simulink model "svm_sim_singleUAS"  (Simulink 8.6)
settings: Solver=ode1  StartTime=0.0  StopTime=svm.tsim  FixedStep=uavsim.svm.tsample_model  RelTol=1e-6
values from neighbouring files (symbols this model uses):
  My_3D = ([eye(6) -eye(6)])    [svm_buildLinearControllers.m]    (also in svm_setup.m = [-eye(6) eye(6)])
  turbulence2loadfactors = blkdiag(T_w2nx, T_w2nz)    [svm_buildLinearControllers.m]
  uavsim = loaded.uavsim    [svm_sandbox.m]
undefined symbols (not defined in the file or in its folder): F, Light, MIL, postracking, sigbuilder_block, svm, uavsimblockset_cartesianToAngle
libraries: svm_lib x4, aerolibtransform2 x3, uavsimBlockset_UAV3DInterface x2, aerolibwind2 x1, aerolibgravity2 x1, uavsimBlockset_VectorNorm x1, aerolibanimutils x1
settings Model: Creator=j.bolting  LastModifiedBy=j.bolting
settings SolverCC: AutoInsertRateTranBlk=on
settings DataIOCC: SaveFormat=Dataset  SignalLoggingSaveFormat=Dataset
settings OptimizationCC: ExpressionDepthLimit=128
settings DebuggingCC: UnderspecifiedInitializationDetection=Simplified  MergeDetectMultiDrivingBlocksExec=error  SolverPrmCheckMsg=none  FcnCallInpInsideContextMsg=EnableAllAsError  StateNameClashWarn=none
settings HardwareCC: ProdBitPerPointer=64  ProdLargestAtomicFloat=Float  ProdIntDivRoundTo=Zero  ProdEndianess=LittleEndian  ProdWordSize=64  ProdHWDeviceType=Intel->x86-64 (Windows64)
settings GRTTargetCC: GeneratePreprocessorConditionals=Use local settings  CombineOutputUpdateFcns=on  GRTInterface=off
settings ConfigComp: CovModelRefEnable=off

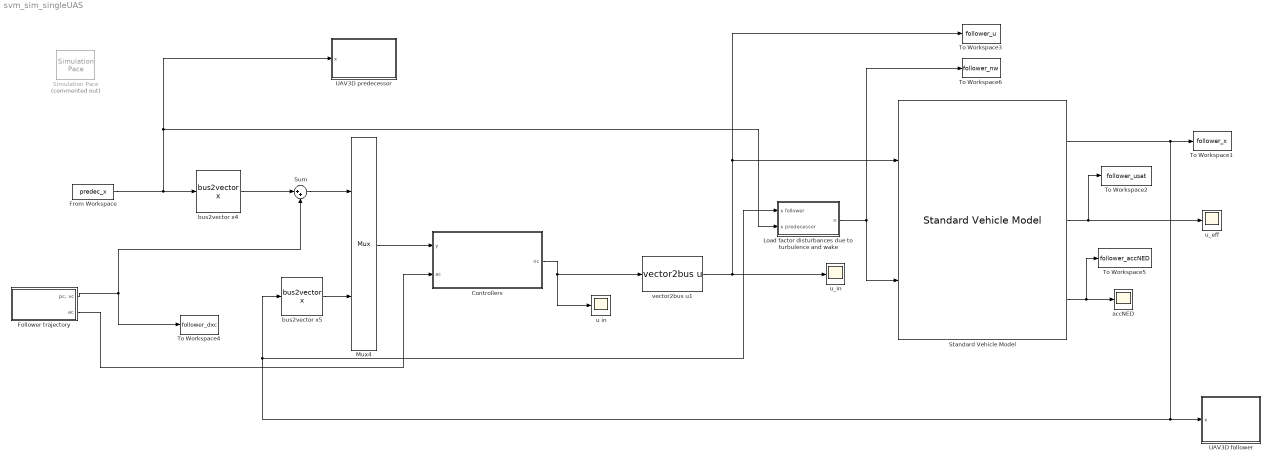
== system svm_sim_singleUAS ==
  Controllers : Subsystem
  Follower trajectory : Subsystem
  From Workspace : FromWorkspace  VariableName=predec_x  OutDataTypeStr=Bus: svm_bus_x
  Load factor disturbances due to turbulence and wake : Subsystem  AncestorBlock=svm_lib/Load factor disturbances due to turbulence
  Mux4 : Mux  Inputs=2
  Simulation Pace : aerolibanimutils/Simulation Pace  Commented=on  SimulationPace=1  SleepMode=MATLAB Thread  OutputPaceError=on  SampleTime=-1
      settings: AttributesFormatString=%<SimulationPace> sec/sec
  Standard Vehicle Model : svm_lib/Standard Vehicle Model  mask_p0_NED=svm.p0  mask_v0_NED=svm.v0
  Sum : Sum  Inputs=|++
  To Workspace1 : ToWorkspace  VariableName=follower_x  SaveFormat=Timeseries  SampleTime=-1
  To Workspace2 : ToWorkspace  VariableName=follower_usat  SaveFormat=Timeseries  SampleTime=-1
  To Workspace3 : ToWorkspace  VariableName=follower_u  SaveFormat=Timeseries  SampleTime=-1
  To Workspace4 : ToWorkspace  VariableName=follower_dxc  SaveFormat=Timeseries  SampleTime=-1
  To Workspace5 : ToWorkspace  VariableName=follower_accNED  SaveFormat=Timeseries  SampleTime=-1
  To Workspace6 : ToWorkspace  VariableName=follower_nw  SaveFormat=Timeseries  SampleTime=-1
  UAV3D follower : Subsystem
  UAV3D predecessor : Subsystem
  accNED : Scope
  bus2vector x4 : svm_lib/bus2vector x
  bus2vector x5 : svm_lib/bus2vector x
  u in : Scope
  u_eff : Scope
  u_in : Scope
  vector2bus u1 : svm_lib/vector2bus u
  wires:
  Standard Vehicle Model/1 -> UAV3D follower/1(x), bus2vector x5/1, Load factor disturbances due to turbulence and wake/1(x follower), To Workspace1/1
  bus2vector x4/1 -> Sum/1
  bus2vector x5/1 -> Mux4/2
  vector2bus u1/1 -> To Workspace3/1, Standard Vehicle Model/1, u_in/1
  From Workspace/1 -> bus2vector x4/1, Load factor disturbances due to turbulence and wake/2(x predecessor), UAV3D predecessor/1(x)
  Controllers/1(nc) -> vector2bus u1/1, u in/1
  Mux4/1 -> Controllers/1(y)
  Load factor disturbances due to turbulence and wake/1(n) -> Standard Vehicle Model/2, To Workspace6/1
  Standard Vehicle Model/2 -> u_eff/1, To Workspace2/1
  Standard Vehicle Model/3 -> accNED/1, To Workspace5/1
  Sum/1 -> Mux4/1
  Follower trajectory/1("pc, vc") -> To Workspace4/1, Sum/2
  Follower trajectory/2(ac) -> Controllers/2(ac)

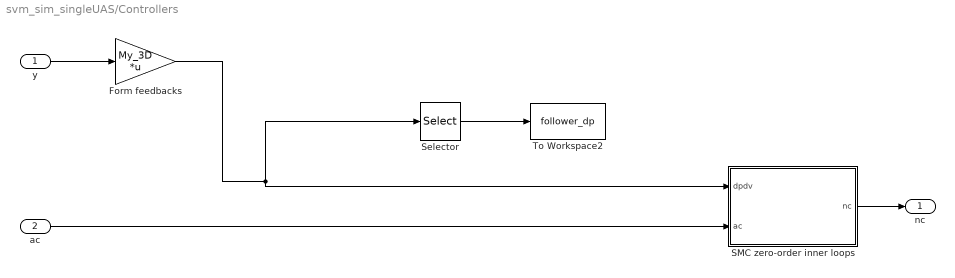
== system svm_sim_singleUAS/Controllers ==
  y : Inport
  ac : Inport  Port=2
  Form feedbacks : Gain  Gain=My_3D  Multiplication=Matrix(K*u)
  SMC zero-order inner loops : Subsystem
  Selector : Selector  InputPortWidth=6  IndexOptions=Index vector (dialog)  Indices=1:3  OutputSizes=1
  To Workspace2 : ToWorkspace  VariableName=follower_dp  SaveFormat=Timeseries  SampleTime=-1
  nc : Outport
  wires:
  SMC zero-order inner loops/1(nc) -> nc/1
  y/1 -> Form feedbacks/1
  Form feedbacks/1 -> Selector/1, SMC zero-order inner loops/1(dpdv)
  ac/1 -> SMC zero-order inner loops/2(ac)
  Selector/1 -> To Workspace2/1

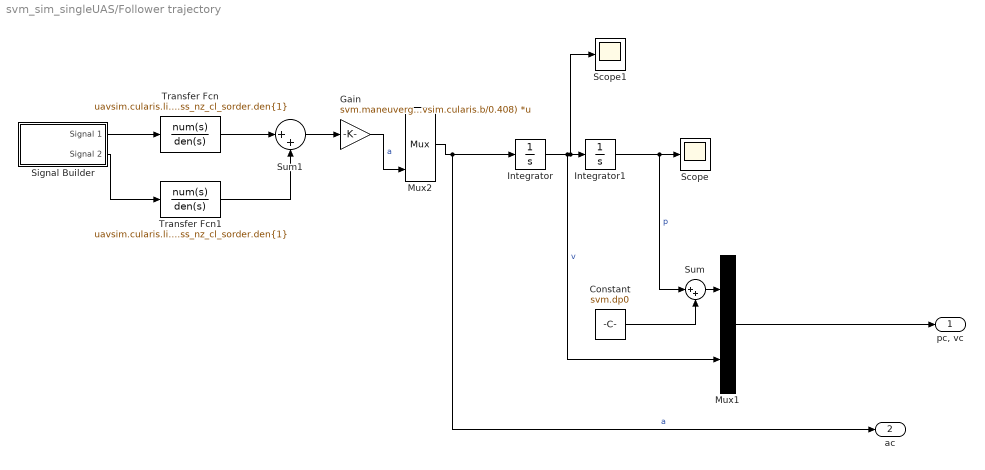
== system svm_sim_singleUAS/Follower trajectory ==
  Constant : Constant  Value=svm.dp0
  Gain : Gain  Gain=svm.maneuvergain*4*(1*uavsim.cularis.b/0.408)  Multiplication=Matrix(K*u)
  Integrator : Integrator
  Integrator1 : Integrator
  Mux1 : Mux  Inputs=2
  Mux2 : Mux  Inputs=3
  Scope : Scope
  Scope1 : Scope
  Signal Builder : Subsystem  Tag=STV Subsys  LoadFcn=sigbuilder_block('load');  StartFcn=sigbuilder_block('start');  StopFcn=sigbuilder_block('stop');  ClipboardFcn=sigbuilder_block('clipboard');  mask(Sigbuilder block){}
      mask help: Simulink:masks:SigbuilderBlock_MD
      mask init:
      | if ~strcmp(get_param(bdroot(gcbh),'SimulationStatus'),'stopped') tuvar = sigbuilder_block('maskInit'); end
      settings: CopyFcn=sigbuilder_block('copy');  DeleteFcn=sigbuilder_block('delete');  ModelCloseFcn=sigbuilder_block('modelClose');  PreSaveFcn=sigbuilder_block('preSave');  PauseFcn=sigbuilder_block('pause');  ContinueFcn=sigbuilder_block('continue');  NameChangeFcn=sigbuilder_block('namechange');  OpenFcn=sigbuilder_block('open',[219.6 199.2 768.6 400.2 ]);  CloseFcn=sigbuilder_block('close');
      mask Display: plot(0, 0, 100, 100,[2, 2, 32, 32, 2], [68, 8, 8, 68, 68],[32, 2], [38, 38], [32, 19, 2],[53, 60, 44], [32, 17, 17, 2],[16, 16, 31, 31]);txt = getActiveGroup(gcbh);text(2, 100, txt,'verticalAlignment', 'top');
  Sum : Sum  Inputs=|++
  Sum1 : Sum  Inputs=|++
  Transfer Fcn : TransferFcn  Numerator=uavsim.cularis.linearModels.eulers.ss_nz_cl_sorder.num{1}  Denominator=uavsim.cularis.linearModels.eulers.ss_nz_cl_sorder.den{1}
  Transfer Fcn1 : TransferFcn  Numerator=uavsim.cularis.linearModels.eulers.ss_nz_cl_sorder.num{1}  Denominator=uavsim.cularis.linearModels.eulers.ss_nz_cl_sorder.den{1}
  "pc, vc" : Outport
  ac : Outport  Port=2
  wires:
  Mux1/1 -> "pc, vc"/1
  Signal Builder/1(Signal 1) -> Transfer Fcn/1
  Signal Builder/2(Signal 2) -> Transfer Fcn1/1
  Sum1/1 -> Gain/1
  Transfer Fcn/1 -> Sum1/1
  Transfer Fcn1/1 -> Sum1/2
  Mux2/1 -> ac/1, Integrator/1  "a"
  Integrator/1 -> Mux1/2, Scope1/1, Integrator1/1  "v"
  Integrator1/1 -> Sum/1, Scope/1  "p"
  Sum/1 -> Mux1/1
  Constant/1 -> Sum/2
  Gain/1 -> Mux2/3  "a"

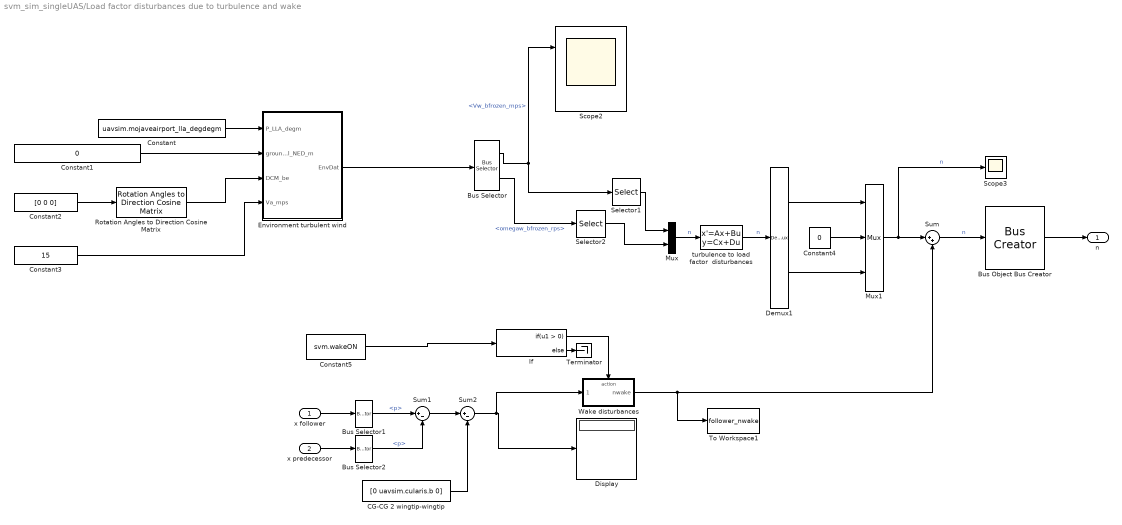
== system svm_sim_singleUAS/Load factor disturbances due to turbulence and wake ==
  x follower : Inport  OutDataTypeStr=Bus: svm_bus_x
  x predecessor : Inport  Port=2  OutDataTypeStr=Bus: svm_bus_x
  Bus Selector : BusSelector  OutputSignals=Vw_bfrozen_mps,omegaw_bfrozen_rps
  Bus Selector1 : BusSelector  OutputSignals=p
  Bus Selector2 : BusSelector  OutputSignals=p
  Bus Object Bus Creator : BusCreator  Inputs=1  OutDataTypeStr=Bus: svm_bus_u  mask(BUS OBJECT Bus Creator){busType=Bus: svm_bus_u}
      mask prompts: busType "Bus Type"
      mask help:
      | Provides users the cabability to painlessly, instantly customize bus creators of output data type 'Bus:' by selecting the bus object type from a drop down menu dynamically populated by bus objects in the workspace.
      |
      | After pressing the "Apply Selection" button signal lines into the creator are populated and named with the elements in the chosen bus saving the user from having to recall and fill out signal line names.
      |
      | NOTE that when copying a Bus Object Bus Creator from your locked Library the link to the Library is automatically broken. This saves the user from having to Unlock Links To Library (From the Library menu.), Disable Link and finally Break Link (Both from the Model menu.) for every placed instance of the block.
      settings: AttributesFormatString=%<OutDataTypeStr>  CopyFcn=set_param(gcb, 'LinkStatus', 'none')
      mask TypeOptions busType: Bus: Acceleration | Bus: Aero | Bus: Airframe | Bus: Attitude | Bus: CMD | Bus: Environment | Bus: FlightGearData | Bus: Kinematics | Bus: Position | Bus: RotationalAcceleration | Bus: RotationalVelocity | Bus: Velocity | Bus: svm_bus_d_exo | Bus: svm_bus_u | Bus: svm_bus_x | Bus: svm_bus_xi
      mask Callback busType:
      | % Using variable names terminated with "_BOBC" to lessen the chances of
      | % collisions with existing workspace variables.
      | 
      | % Get the current block handle and mask handle.
      | handleCreator_BOBC = gcbh;
      | maskObj_BOBC       = Simulink.Mask.get(gcb);
      | 
      | % Get a list of variables in the workspace in order to search for the '1x1
      | % Bus' types.
      | wsVars_BOBC = whos;
      | 
      | % Reset the 'TypeOptions' bus list in case some '1x1 Bus' types have been
      | % deleted from or added to the workspace.
      | maskObj_BOBC.Parameters.TypeOptions = {'<empty>'};
      | 
      | % Reset the bus count.
      | busCount_BOBC = 0;
      | 
      | for index_BOBC = 1:length(wsVars_BOBC)
      | 
      |    % If the variable is a bus object...
      |    if strcmp(wsVars_BOBC(index_BOBC).class, 'Simulink.Bus')
      | 
      |       busCount_BOBC = busCount_BOBC + 1;
      | 
      |       % ... add it to the TypeOptions of the mask.
      |       maskObj_BOBC.Parameters.TypeOptions(busCount_BOBC) = ...
      |                                                            ...
      |                                  {['Bus: ', wsVars_BOBC(index_BOBC).name]};
      |    end
      | end
      | 
      | if busCount_BOBC == 0
      | 
      |    % If there are NO bus objects in the workspace then provide a warning
      |    % popup...
      |    warndlg('There are currently no bus objects in the workspace - you have no use for this block. Use a normal Bus Creator instead.')
      | 
      |    % ... and do nothing.
      | elseif ~strcmp(get_param(handleCreator_BOBC, 'OutDataTypeStr'), 'Inherit: auto')
      | 
      |    % If the currently selected bus data type ('OutDataTypeStr') is not
      |    % 'Inherit: auto' (i.e., if we are reopening the mask.) then get the
      |    % current 'OutDataTypeStr' and 'maskVal.' ('maskVal' is the selected
      |    % 'TypeOptions' list member.)
      |    outDatStr_BOBC = get_param(handleCreator_BOBC, 'OutDataTypeStr');
      |    maskVal_BOBC   = get_param(handleCreator_BOBC, 'MaskValues');
      | 
      |    if ~strcmp(outDatStr_BOBC, maskVal_BOBC{1})
      | 
      |       % Upon re-opening the mask if the default 'TypeOptions' list member
      |       % (The first one.) contained in 'maskVal' does not match the
      |       % currently selected bus data type ('OutDataTypeStr') then set the
      |       % 'TypeOptions' list member to the selected bus data type. (Cuts down
      |       % on confusion to have the displayed list member match the selected
      |       % bus data type rather than the first entry.)
      |       set_param(handleCreator_BOBC, 'MaskValues', {outDatStr_BOBC});
      |    end
      | end
      | 
      | % Clean up the workspace.
      | clear  handleCreator_BOBC  maskObj_BOBC     wsVars_BOBC ...
      |             busCount_BOBC    index_BOBC  outDatStr_BOBC ...
      |              maskVal_BOBC
      mask DialogControl applyMOCBSelection Prompt: Apply Selection
      mask DialogControl applyMOCBSelection Callback:
      | % Using variable names terminated with "_BOBC" to lessen the chances of
      | % collisions with existing workspace variables.
      | 
      | % Get the current block, current block handle and mask handle.
      | currentBlock_BOBC  = gcb;
      | handleCreator_BOBC = gcbh;
      | 
      | % Get the desired bus type...
      | desiredBusType_BOBC = get_param(handleCreator_BOBC, 'busType');
      | 
      | % ... and set the 'OutDataTypeStr' to it.
      | set_param(handleCreator_BOBC, 'OutDataTypeStr', desiredBusType_BOBC);
      | 
      | %% First delete any existing lines on the port.
      | % Get the line handles.
      | lh_BOBC = get_param(handleCreator_BOBC, 'LineHandles');
      | 
      | % If any lines exist (Non- -1 line handles.), delete them and start over.
      | if max(lh_BOBC.Inport > 0)
      | 
      |    for index_BOBC = 1:length(lh_BOBC.Inport)
      | 
      |       if lh_BOBC.Inport(index_BOBC) > 0
      | 
      |          delete_line(lh_BOBC.Inport(index_BOBC))
      |       end
      |    end
      | end
      | 
      | %% Then work on adding new lines.
      | 
      | % Get the block path for 'add_line' function.
      | blockPath_BOBC = get_param(handleCreator_BOBC, 'Parent');
      | 
      | % Get the newly selected bus type ('OutDataTypeStr')...
      | mocbBusType_BOBC = get_param(currentBlock_BOBC, 'OutDataTypeStr');
      | 
      | % ... and parse off "Bus: " so the string of the desired bus contained in
      | % 'OutDataTypeStr' matches the raw workspace bus names.
      | mocbBusType_BOBC = mocbBusType_BOBC(6:end);
      | 
      | % Then evaluate the string containing the workspace bus name which will
      | % load the desired bus parameters.
      | busParams_BOBC = eval(mocbBusType_BOBC);
      | 
      | % From the parameters grab the number of lines to add.
      | numLines_BOBC = length(busParams_BOBC.Elements);
      | 
      | % Set the number of inputs of the masked bus creator to the number of lines
      | % to add.
      | set_param(handleCreator_BOBC, 'Inputs', num2str(numLines_BOBC));
      | 
      | % Get (Inputs.) port handles so we can grab the positions of them.
      | ph_BOBC = get_param(handleCreator_BOBC, 'PortHandles');
      | 
      | for index_BOBC = 1:numLines_BOBC
      | 
      |    % Get the position of input port number 'index_BOBC'.
      |    portPos_BOBC = get_param(ph_BOBC.Inport(index_BOBC), 'Position');
      | 
      |    % Add a line from 50 pixels left of the port position to the port
      |    % position. (This must be done because it's the lines that get named,
      |    % not the port positions.)
      |    portLine_BOBC = add_line(blockPath_BOBC, [portPos_BOBC - [50 0]; portPos_BOBC]);
      | 
      |    % Rename the new line to the bus 'index_BOBC-st/nd/rd/th' element name.
      |    set_param(portLine_BOBC, 'Name', busParams_BOBC.Elements(index_BOBC).Name)
      | end
      | 
      | %% Cleanup the workspace.
      | clear    currentBlock_BOBC  handleCreator_BOBC      index_BOBC ...
      |        desiredBusType_BOBC             lh_BOBC  blockPath_BOBC ...
      |           mocbBusType_BOBC      busParams_BOBC   numLines_BOBC ...
      |                    ph_BOBC        portPos_BOBC   portLine_BOBC
  CG-CG 2 wingtip-wingtip : Constant  Value=[0 uavsim.cularis.b 0]
  Constant : Constant  Value=uavsim.mojaveairport_lla_degdegm
  Constant1 : Constant  Value=0
  Constant2 : Constant  Value=[0 0 0]
  Constant3 : Constant  Value=15
  Constant4 : Constant  Value=0
  Constant5 : Constant  Value=svm.wakeON
  Demux1 : Demux  Outputs=2
  Display : Display
  Environment turbulent wind : Subsystem  AncestorBlock=uavsimBlockset_Environment_turbulentWind/Environment turbulent wind  mask{mask_constantwind_NED_mps=svm.ambientWind, mask_wingspan=uavsim.cularis.b, mask_windON=svm.ambientWindOn, mask_turbulenceON=svm.turbulenceOn}
      mask prompts: mask_constantwind_NED_mps "Ambient, i.e. constant wind vector [m/s], NED frame"; mask_wingspan "Aircraft wingspan"; mask_windON "Ambient wind ON?"; mask_turbulenceON "Turbulence ON?"
  If : If
  Mux : Mux  Inputs=2
  Mux1 : Mux  Inputs=3
  Rotation Angles to Direction Cosine Matrix : aerolibtransform2/Rotation Angles to Direction Cosine Matrix  rotationOrder=ZYX
  Scope2 : Scope  NumInputPorts=2
  Scope3 : Scope
  Selector1 : Selector  InputPortWidth=3  IndexOptions=Index vector (dialog)  Indices=[1 3]  OutputSizes=1
  Selector2 : Selector  InputPortWidth=3  IndexOptions=Index vector (dialog)  Indices=2  OutputSizes=1
  Sum : Sum  Inputs=|++
  Sum1 : Sum  Inputs=|+-
  Sum2 : Sum  Inputs=|+-
  Terminator : Terminator
  To Workspace1 : ToWorkspace  VariableName=follower_nwake  SaveFormat=Timeseries  SampleTime=-1
  Wake disturbances : Subsystem  TreatAsAtomicUnit=on
  turbulence to load factor  disturbances : StateSpace  A=turbulence2loadfactors.a  B=turbulence2loadfactors.b  C=turbulence2loadfactors.c  D=turbulence2loadfactors.d  X0=0
  n : Outport
  wires:
  Constant4/1 -> Mux1/2
  Demux1/2 -> Mux1/3
  Mux1/1 -> Sum/1, Scope3/1  "n"
  Selector2/1 -> Mux/2
  Constant2/1 -> Rotation Angles to Direction Cosine Matrix/1
  turbulence to load factor  disturbances/1 -> Demux1/1  "n"
  Constant1/1 -> Environment turbulent wind/2(groundlevel_NED_m)
  Demux1/1 -> Mux1/1
  Constant/1 -> Environment turbulent wind/1(P_LLA_degm)
  Bus Selector/1 -> Scope2/1, Selector1/1  "<Vw_bfrozen_mps>"
  Rotation Angles to Direction Cosine Matrix/1 -> Environment turbulent wind/3(DCM_be)
  Bus Selector/2 -> Selector2/1  "<omegaw_bfrozen_rps>"
  Environment turbulent wind/1(EnvDat) -> Bus Selector/1
  Constant3/1 -> Environment turbulent wind/4(Va_mps)
  Bus Object Bus Creator/1 -> n/1
  Mux/1 -> turbulence to load factor  disturbances/1  "n"
  Selector1/1 -> Mux/1
  If/1 -> Wake disturbances/Action
  Constant5/1 -> If/1
  If/2 -> Terminator/1
  Wake disturbances/1(nwake) -> Sum/2, To Workspace1/1
  x follower/1 -> Bus Selector1/1
  x predecessor/1 -> Bus Selector2/1
  Bus Selector1/1 -> Sum1/1  "<p>"
  Bus Selector2/1 -> Sum1/2  "<p>"
  Sum2/1 -> Wake disturbances/1(dp_wingtips), Display/1
  CG-CG 2 wingtip-wingtip/1 -> Sum2/2
  Sum1/1 -> Sum2/1
  Sum/1 -> Bus Object Bus Creator/1  "n"

== system svm_sim_singleUAS/UAV3D follower ==
  x : Inport
  Bus Selector5 : BusSelector  OutputSignals=p,v
  Rate Transition10 : RateTransition  OutPortSampleTime=uavsim.svm.tsample_uav3d
  Rate Transition9 : RateTransition  OutPortSampleTime=uavsim.svm.tsample_uav3d
  Vehicle ID2 : Constant  Value=2
  Visualize NED position2 : Subsystem  AncestorBlock=formationFlyingBlockset/Visualize leader  TreatAsAtomicUnit=on  SystemSampleTime=uavsim.svm.tsample_uav3d  mask{mask_3dmodel=1}
      mask prompts: mask_3dmodel "3D model"
      mask TypeOptions mask_3dmodel: 0 | 1 | 2 | 3
  wires:
  x/1 -> Bus Selector5/1
  Bus Selector5/2 -> Rate Transition10/1  "<v>"
  Vehicle ID2/1 -> Visualize NED position2/3(ID)
  Bus Selector5/1 -> Rate Transition9/1  "<p>"
  Rate Transition10/1 -> Visualize NED position2/2(v_NED_mps)
  Rate Transition9/1 -> Visualize NED position2/1(p_NED_m)

== system svm_sim_singleUAS/UAV3D predecessor ==
  x : Inport
  Bus Selector1 : BusSelector  OutputSignals=p,v
  Constant5 : Constant
  Rate Transition5 : RateTransition  OutPortSampleTime=uavsim.svm.tsample_uav3d
  Rate Transition6 : RateTransition  OutPortSampleTime=uavsim.svm.tsample_uav3d
  Visualize NED position1 : Subsystem  AncestorBlock=formationFlyingBlockset/Visualize leader  TreatAsAtomicUnit=on  SystemSampleTime=uavsim.svm.tsample_uav3d  mask{mask_3dmodel=1}
      mask prompts: mask_3dmodel "3D model"
      mask TypeOptions mask_3dmodel: 0 | 1 | 2 | 3
  wires:
  x/1 -> Bus Selector1/1
  Rate Transition5/1 -> Visualize NED position1/1(p_NED_m)
  Constant5/1 -> Visualize NED position1/3(ID)
  Rate Transition6/1 -> Visualize NED position1/2(v_NED_mps)
  Bus Selector1/1 -> Rate Transition5/1  "<p>"
  Bus Selector1/2 -> Rate Transition6/1  "<v>"

== system svm_sim_singleUAS/Controllers/SMC zero-order inner loops ==
  dpdv : Inport
  ac : Inport  Port=2
  CSMC : Subsystem  Commented=on  AncestorBlock=svm_lib/SMC-directforce
  DSMC : Subsystem  AncestorBlock=svm_lib/SMC-directforce
  nc : Outport
  wires:
  DSMC/1(nc) -> nc/1
  dpdv/1 -> CSMC/1(dpdv), DSMC/1(dpdv)
  ac/1 -> DSMC/2(ac)

== system svm_sim_singleUAS/Follower trajectory/Signal Builder ==
  Demux : Demux  Tag=STV Demux  Outputs=2
  FromWs : FromWorkspace  Tag=STV FromWs  VariableName=tuvar  SampleTime=0  SigBuilderData=DataTag0  VnvData=DataTag1
      SigBuilderData=|
      | common.afterFinalStr = 'Extrapolate'
      | common.sampleTime = 0
      | dataSet.timeRange = [0 10]
      | dataSet.name = 'Group 1'
      | sbobj.Groups.Name = 'Group 1'
      | sbobj.Groups.Signals(1).Name = 'Signal 1'
      | sbobj.Groups.Signals(1).XData = [0 5 5 6.02 6.02 10]
      | sbobj.Groups.Signals(1).YData = [0 0 -0.1 -0.1 0 0]
      | sbobj.Groups.Signals(2).Name = 'Signal 2'
      | sbobj.Groups.Signals(2).XData = [0 6 6 7.02 7.02 10]
      | sbobj.Groups.Signals(2).YData = [0 0 0.1 0.1 0 0]
  Signal 1 : Outport  Tag=STV Outport
  Signal 2 : Outport  Tag=STV Outport  Port=2
  wires:
  Demux/1 -> Signal 1/1
  FromWs/1 -> Demux/1
  Demux/2 -> Signal 2/1

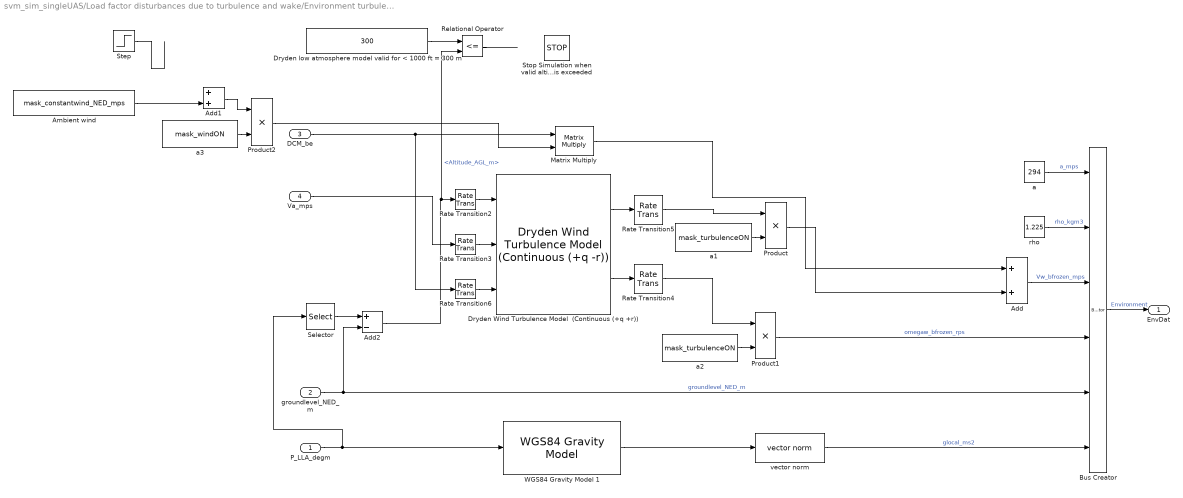
== system svm_sim_singleUAS/Load factor disturbances due to turbulence and wake/Environment turbulent wind ==
  P_LLA_degm : Inport
  groundlevel_NED_m : Inport  Port=2
  DCM_be : Inport  Port=3
  Va_mps : Inport  Port=4
  Add : Sum
  Add1 : Sum
  Add2 : Sum  Inputs=+-
  Ambient wind : Constant  Value=mask_constantwind_NED_mps
  Bus Creator : BusCreator  Inputs=6  OutDataTypeStr=Bus: Environment  NonVirtualBus=on
  Dryden Wind Turbulence Model  (Continuous (+q +r)) : aerolibwind2/Dryden Wind Turbulence Model  (Continuous (+q -r))  units=Metric (MKS)  spec=MIL-F-8785C  model=Discrete Dryden (+q -r)  W20=norm(mask_constantwind_NED_mps)  Wdeg=rad2deg(uavsimblockset_cartesianToAngle(mask_constantwind_NED_mps(1), mask_constantwind_NED_mps(2)))  TurbProb=10^-2 - Light  L_high=533.4  Wingspan=mask_wingspan  ts=uavsim.svm.tsample_dryden  Seed=eval(svm.turbulenceseed)  T_on=on
  Dryden low atmosphere model valid for < 1000 ft = 300 m : Constant  Value=300
  Matrix Multiply : Product  Multiplication=Matrix(*)
  Product : Product  RndMeth=Zero
  Product1 : Product  RndMeth=Zero
  Product2 : Product  RndMeth=Zero
  Rate Transition2 : RateTransition  OutPortSampleTime=uavsim.svm.tsample_dryden
  Rate Transition3 : RateTransition  OutPortSampleTime=uavsim.svm.tsample_dryden
  Rate Transition4 : RateTransition  OutPortSampleTime=0
  Rate Transition5 : RateTransition  OutPortSampleTime=0
  Rate Transition6 : RateTransition  OutPortSampleTime=uavsim.svm.tsample_dryden
  Relational Operator : RelationalOperator  Operator=<=  OutDataTypeStr=boolean
  Selector : Selector  InputPortWidth=3  IndexOptions=Index vector (dialog)  Indices=3  OutputSizes=1
  Step : Step  Time=10  After=[0 0 1]  SampleTime=0
  Stop Simulation when valid altitude is exceeded : Stop
  WGS84 Gravity Model 1 : aerolibgravity2/WGS84 Gravity Model   model=WGS84 Taylor Series  units=Metric (MKS)  no_atmos=on  precessing=on  jd_loc=off  month=October  day=10  year=2004  no_centrifugal=on  action=Warning
  a : Constant  Value=294
  a1 : Constant  Value=mask_turbulenceON
  a2 : Constant  Value=mask_turbulenceON
  a3 : Constant  Value=mask_windON
  "rho " : Constant  Value=1.225
  vector norm : uavsimBlockset_VectorNorm/vector norm
  EnvDat : Outport  OutDataTypeStr=Bus: Environment
  wires:
  Rate Transition6/1 -> Dryden Wind Turbulence Model  (Continuous (+q +r))/3
  Rate Transition3/1 -> Dryden Wind Turbulence Model  (Continuous (+q +r))/2
  Rate Transition2/1 -> Dryden Wind Turbulence Model  (Continuous (+q +r))/1
  Selector/1 -> Add2/1
  Rate Transition5/1 -> Product/1
  Rate Transition4/1 -> Product1/1
  Matrix Multiply/1 -> Add/1
  Dryden Wind Turbulence Model  (Continuous (+q +r))/1 -> Rate Transition5/1
  Ambient wind/1 -> Add1/2
  DCM_be/1 -> Rate Transition6/1, Matrix Multiply/1
  Va_mps/1 -> Rate Transition3/1
  Add2/1 -> Relational Operator/2, Rate Transition2/1  "<Altitude_AGL_m>"
  vector norm/1 -> Bus Creator/6  "glocal_ms2"
  Add/1 -> Bus Creator/3  "Vw_bfrozen_mps"
  a/1 -> Bus Creator/1  "a_mps"
  "rho "/1 -> Bus Creator/2  "rho_kgm3"
  Bus Creator/1 -> EnvDat/1  "Environment"
  WGS84 Gravity Model 1/1 -> vector norm/1
  groundlevel_NED_m/1 -> Bus Creator/5, Add2/2  "groundlevel_NED_m"
  P_LLA_degm/1 -> Selector/1, WGS84 Gravity Model 1/1
  Dryden Wind Turbulence Model  (Continuous (+q +r))/2 -> Rate Transition4/1
  Product/1 -> Add/2
  a1/1 -> Product/2
  a2/1 -> Product1/2
  Product1/1 -> Bus Creator/4  "omegaw_bfrozen_rps"
  Dryden low atmosphere model valid for < 1000 ft = 300 m/1 -> Relational Operator/1
  Relational Operator/1 -> ?
  a3/1 -> Product2/2
  Product2/1 -> Matrix Multiply/2
  Add1/1 -> Product2/1
  Step/1 -> ?

== system svm_sim_singleUAS/Load factor disturbances due to turbulence and wake/Wake disturbances ==
  dp_wingtips : Inport
  Action Port : ActionPort  ActionType=then
  MATLAB Function : MATLAB Function  TreatAsAtomicUnit=on
  nwake : Outport
  wires:
  dp_wingtips/1 -> MATLAB Function/1(dp)
  MATLAB Function/1(nwake) -> nwake/1

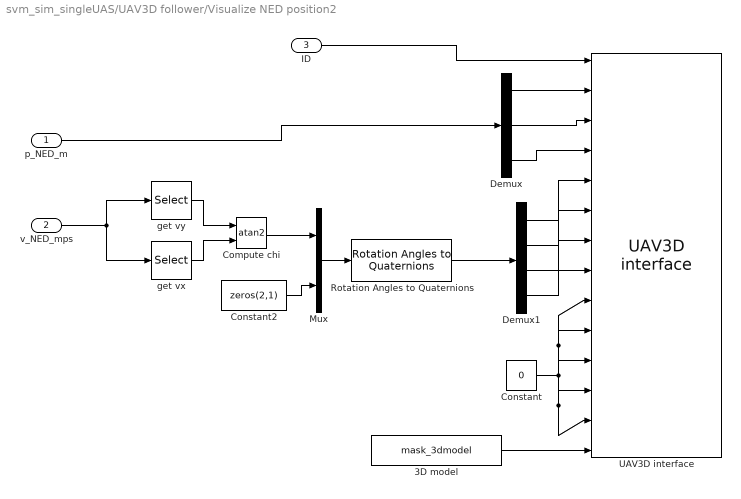
== system svm_sim_singleUAS/UAV3D follower/Visualize NED position2 ==
  p_NED_m : Inport
  v_NED_mps : Inport  Port=2
  ID : Inport  Port=3
  3D model : Constant  Value=mask_3dmodel
  Compute chi : Trigonometry  Operator=atan2
  Constant : Constant  Value=0
  Constant2 : Constant  Value=zeros(2,1)
  Demux : Demux  Outputs=3
  Demux1 : Demux
  Mux : Mux  Inputs=2
  Rotation Angles to Quaternions : aerolibtransform2/Rotation Angles to Quaternions  rotationOrder=ZYX
  UAV3D interface : uavsimBlockset_UAV3DInterface/UAV3D interface  ip='localhost'  udpport=4445
  get vx : Selector  InputPortWidth=3  IndexOptions=Index vector (dialog)  Indices=1  OutputSizes=1
  get vy : Selector  InputPortWidth=3  IndexOptions=Index vector (dialog)  Indices=2  OutputSizes=1
  wires:
  Demux/1 -> UAV3D interface/2
  Demux/2 -> UAV3D interface/3
  Demux/3 -> UAV3D interface/4
  Demux1/1 -> UAV3D interface/5
  Demux1/2 -> UAV3D interface/6
  Demux1/4 -> UAV3D interface/8
  p_NED_m/1 -> Demux/1
  get vy/1 -> Compute chi/1
  get vx/1 -> Compute chi/2
  v_NED_mps/1 -> get vy/1, get vx/1
  Constant2/1 -> Mux/2
  Mux/1 -> Rotation Angles to Quaternions/1
  Rotation Angles to Quaternions/1 -> Demux1/1
  Compute chi/1 -> Mux/1
  Demux1/3 -> UAV3D interface/7
  Constant/1 -> UAV3D interface/13, UAV3D interface/12, UAV3D interface/11, UAV3D interface/10, UAV3D interface/9
  ID/1 -> UAV3D interface/1
  3D model/1 -> UAV3D interface/14

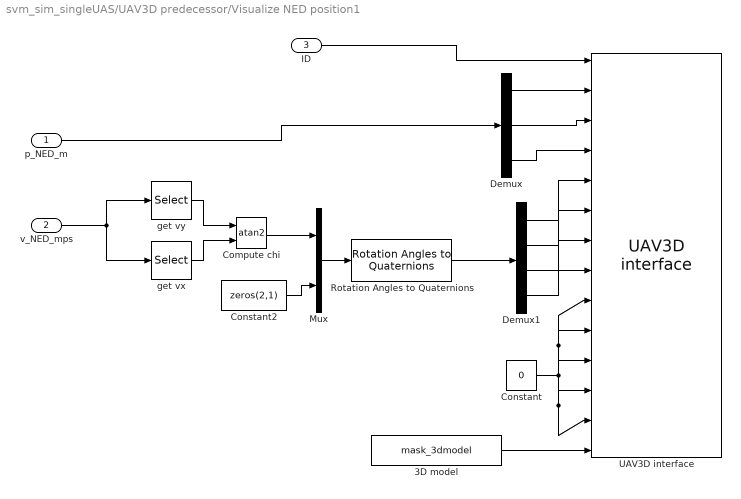
== system svm_sim_singleUAS/UAV3D predecessor/Visualize NED position1 ==
  p_NED_m : Inport
  v_NED_mps : Inport  Port=2
  ID : Inport  Port=3
  3D model : Constant  Value=mask_3dmodel
  Compute chi : Trigonometry  Operator=atan2
  Constant : Constant  Value=0
  Constant2 : Constant  Value=zeros(2,1)
  Demux : Demux  Outputs=3
  Demux1 : Demux
  Mux : Mux  Inputs=2
  Rotation Angles to Quaternions : aerolibtransform2/Rotation Angles to Quaternions  rotationOrder=ZYX
  UAV3D interface : uavsimBlockset_UAV3DInterface/UAV3D interface  ip='localhost'  udpport=4445
  get vx : Selector  InputPortWidth=3  IndexOptions=Index vector (dialog)  Indices=1  OutputSizes=1
  get vy : Selector  InputPortWidth=3  IndexOptions=Index vector (dialog)  Indices=2  OutputSizes=1
  wires:
  Demux/1 -> UAV3D interface/2
  Demux/2 -> UAV3D interface/3
  Demux/3 -> UAV3D interface/4
  Demux1/1 -> UAV3D interface/5
  Demux1/2 -> UAV3D interface/6
  Demux1/4 -> UAV3D interface/8
  p_NED_m/1 -> Demux/1
  get vy/1 -> Compute chi/1
  get vx/1 -> Compute chi/2
  v_NED_mps/1 -> get vy/1, get vx/1
  Constant2/1 -> Mux/2
  Mux/1 -> Rotation Angles to Quaternions/1
  Rotation Angles to Quaternions/1 -> Demux1/1
  Compute chi/1 -> Mux/1
  Demux1/3 -> UAV3D interface/7
  Constant/1 -> UAV3D interface/13, UAV3D interface/12, UAV3D interface/11, UAV3D interface/10, UAV3D interface/9
  ID/1 -> UAV3D interface/1
  3D model/1 -> UAV3D interface/14

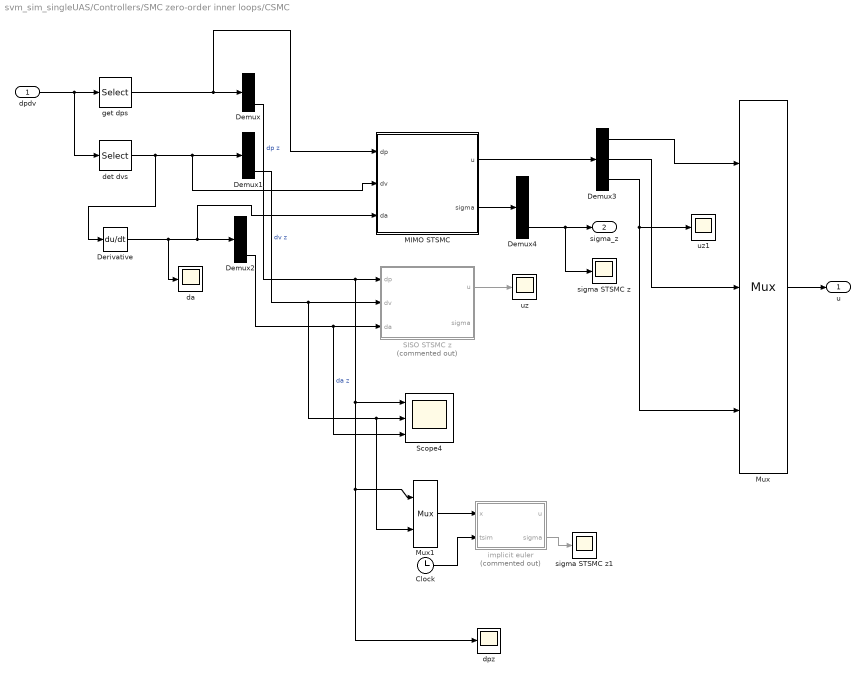
== system svm_sim_singleUAS/Controllers/SMC zero-order inner loops/CSMC ==
  dpdv : Inport
  Clock : Clock
  Demux{,1..4} (5 alike) : Demux  Outputs=3
  Derivative : Derivative
  MIMO STSMC : Subsystem  AncestorBlock=svm_lib/SISO STSMC
  Mux : Mux  Inputs=3
  Mux1 : Mux  Inputs=2
  SISO STSMC z : Subsystem  Commented=on  AncestorBlock=svm_lib/SISO STSMC  mask{mask_k1=-1, mask_k2=-1, mask_lambda=[6; 4; 0], mask_T=postracking.T, mask_U=1}
      mask prompts: mask_k1 "k1"; mask_k2 "k2"; mask_lambda "lambda"; mask_T "Sampling time, zero-order hold"; mask_U "U"
  Scope4 : Scope  NumInputPorts=3
  da : Scope
  det dvs : Selector  InputPortWidth=6  IndexOptions=Index vector (dialog)  Indices=4:6  OutputSizes=1
  dpz : Scope
  get dps : Selector  InputPortWidth=6  IndexOptions=Index vector (dialog)  Indices=1:3  OutputSizes=1
  implicit euler : MATLAB Function  Commented=on  AncestorBlock=svm_lib/implicit euler  TreatAsAtomicUnit=on  SystemSampleTime=postracking.T
  sigma STSMC z : Scope
  sigma STSMC z1 : Scope
  uz : Scope
  uz1 : Scope
  u : Outport
  sigma_z : Outport  Port=2
  wires:
  SISO STSMC z/1(u) -> uz/1
  Demux2/3 -> SISO STSMC z/3(da), Scope4/3  "da z"
  Derivative/1 -> MIMO STSMC/3(da), Demux2/1, da/1
  dpdv/1 -> det dvs/1, get dps/1
  get dps/1 -> MIMO STSMC/1(dp), Demux/1
  det dvs/1 -> MIMO STSMC/2(dv), Demux1/1, Derivative/1
  Mux/1 -> u/1
  Demux1/3 -> SISO STSMC z/2(dv), Mux1/2, Scope4/2  "dv z"
  Demux/3 -> SISO STSMC z/1(dp), Mux1/1, dpz/1, Scope4/1  "dp z"
  Mux1/1 -> implicit euler/1(x)
  Clock/1 -> implicit euler/2(tsim)
  implicit euler/2(sigma) -> sigma STSMC z1/1
  MIMO STSMC/1(u) -> Demux3/1
  Demux3/3 -> Mux/3, uz1/1
  MIMO STSMC/2(sigma) -> Demux4/1
  Demux4/3 -> sigma STSMC z/1, sigma_z/1
  Demux3/2 -> Mux/2
  Demux3/1 -> Mux/1

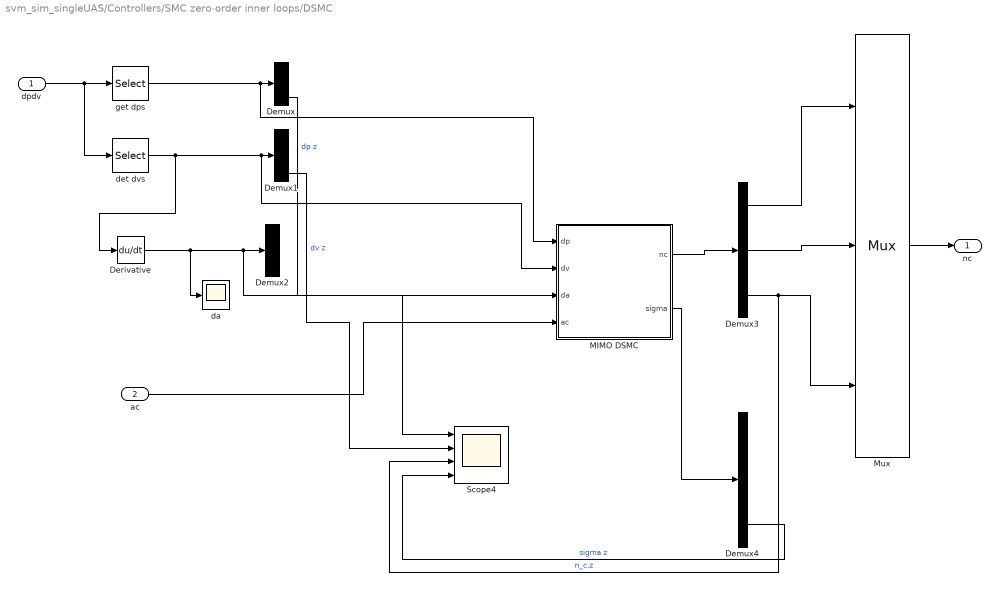
== system svm_sim_singleUAS/Controllers/SMC zero-order inner loops/DSMC ==
  dpdv : Inport
  ac : Inport  Port=2
  Demux{,1..4} (5 alike) : Demux  Outputs=3
  Derivative : Derivative
  MIMO DSMC : Subsystem  AncestorBlock=svm_lib/SISO STSMC
  Mux : Mux  Inputs=3
  Scope4 : Scope  NumInputPorts=4
  da : Scope
  det dvs : Selector  InputPortWidth=6  IndexOptions=Index vector (dialog)  Indices=4:6  OutputSizes=1
  get dps : Selector  InputPortWidth=6  IndexOptions=Index vector (dialog)  Indices=1:3  OutputSizes=1
  nc : Outport
  wires:
  Demux/3 -> Scope4/1  "dp z"
  Demux1/3 -> Scope4/2  "dv z"
  Mux/1 -> nc/1
  get dps/1 -> MIMO DSMC/1(dp), Demux/1
  dpdv/1 -> get dps/1, det dvs/1
  Derivative/1 -> da/1, MIMO DSMC/3(da), Demux2/1
  MIMO DSMC/1(nc) -> Demux3/1
  MIMO DSMC/2(sigma) -> Demux4/1
  Demux3/3 -> Scope4/3, Mux/3  "n_c,z"
  Demux3/2 -> Mux/2
  Demux3/1 -> Mux/1
  det dvs/1 -> Derivative/1, MIMO DSMC/2(dv), Demux1/1
  ac/1 -> MIMO DSMC/4(ac)
  Demux4/3 -> Scope4/4  "sigma z"

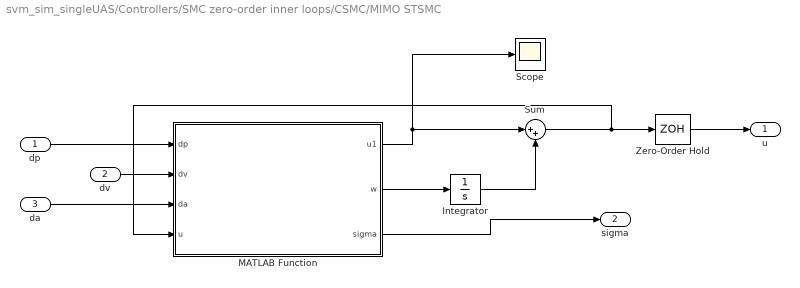
== system svm_sim_singleUAS/Controllers/SMC zero-order inner loops/CSMC/MIMO STSMC ==
  dp : Inport
  dv : Inport  Port=2
  da : Inport  Port=3
  Integrator : Integrator
  MATLAB Function : MATLAB Function  TreatAsAtomicUnit=on
  Scope : Scope
  Sum : Sum  Inputs=|++
  Zero-Order Hold : ZeroOrderHold  SampleTime=postracking.T
  u : Outport
  sigma : Outport  Port=2
  wires:
  da/1 -> MATLAB Function/3(da)
  Sum/1 -> Zero-Order Hold/1, MATLAB Function/4(u)
  Zero-Order Hold/1 -> u/1
  dv/1 -> MATLAB Function/2(dv)
  MATLAB Function/3(sigma) -> sigma/1
  Integrator/1 -> Sum/2
  MATLAB Function/1(u1) -> Sum/1, Scope/1
  MATLAB Function/2(w) -> Integrator/1
  dp/1 -> MATLAB Function/1(dp)

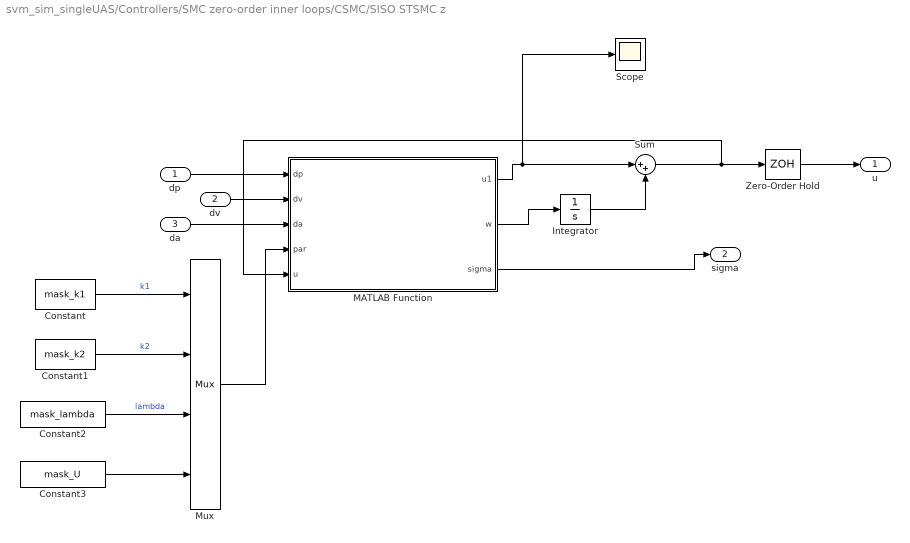
== system svm_sim_singleUAS/Controllers/SMC zero-order inner loops/CSMC/SISO STSMC z ==
  dp : Inport
  dv : Inport  Port=2
  da : Inport  Port=3
  Constant : Constant  Value=mask_k1
  Constant1 : Constant  Value=mask_k2
  Constant2 : Constant  Value=mask_lambda
  Constant3 : Constant  Value=mask_U
  Integrator : Integrator
  MATLAB Function : MATLAB Function  TreatAsAtomicUnit=on
  Mux : Mux
  Scope : Scope
  Sum : Sum  Inputs=|++
  Zero-Order Hold : ZeroOrderHold  SampleTime=mask_T
  u : Outport
  sigma : Outport  Port=2
  wires:
  MATLAB Function/2(w) -> Integrator/1
  MATLAB Function/1(u1) -> Scope/1, Sum/1
  Integrator/1 -> Sum/2
  MATLAB Function/3(sigma) -> sigma/1
  dp/1 -> MATLAB Function/1(dp)
  dv/1 -> MATLAB Function/2(dv)
  Mux/1 -> MATLAB Function/4(par)
  Constant/1 -> Mux/1  "k1"
  Constant1/1 -> Mux/2  "k2"
  Constant2/1 -> Mux/3  "lambda"
  Zero-Order Hold/1 -> u/1
  Constant3/1 -> Mux/4
  Sum/1 -> MATLAB Function/5(u), Zero-Order Hold/1
  da/1 -> MATLAB Function/3(da)

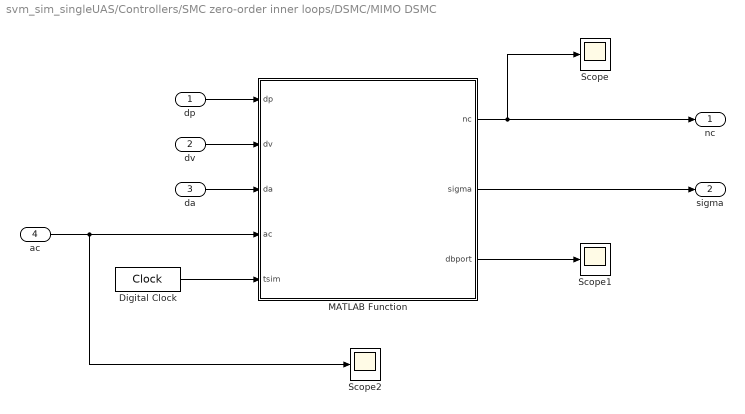
== system svm_sim_singleUAS/Controllers/SMC zero-order inner loops/DSMC/MIMO DSMC ==
  dp : Inport
  dv : Inport  Port=2
  da : Inport  Port=3
  ac : Inport  Port=4
  Digital Clock : DigitalClock  SampleTime=-1
  MATLAB Function : MATLAB Function  TreatAsAtomicUnit=on  SystemSampleTime=postracking.T
  Scope : Scope
  Scope1 : Scope
  Scope2 : Scope
  nc : Outport
  sigma : Outport  Port=2
  wires:
  da/1 -> MATLAB Function/3(da)
  MATLAB Function/1(nc) -> nc/1, Scope/1
  dv/1 -> MATLAB Function/2(dv)
  MATLAB Function/2(sigma) -> sigma/1
  dp/1 -> MATLAB Function/1(dp)
  ac/1 -> Scope2/1, MATLAB Function/4(ac)
  MATLAB Function/3(dbport) -> Scope1/1
  Digital Clock/1 -> MATLAB Function/5(tsim)

== matlab function Controllers/SMC zero-order inner loops/CSMC/SISO STSMC z/MATLAB Function ==
  data: u1 output double; dp input double; dv input double; da input double; par input double; w output double; sigma output double; u input double
function [u1, w, sigma ] = fcn(dp, dv, da, par, u)
coder.extrinsic('blkdiag');
u1 = 0;
sigma = 0;
w = 0;
persistent lastsample;
if isempty(lastsample)
    lastsample.sigma = 0;
end
G = [par(3) par(4) par(5)];
sigma = G * [dp; dv; da];
if sigma > 0
    bp=0;
end
% Discrete approximation of sigmaDot:
sigmaDot = sigma - lastsample.sigma;
lastsample.sigma = sigma;

% Compute controller params in compliance with ACA article:
% Known disturbances:
G_3D = zeros(3,9);
G_3D = blkdiag(G, G, G)
B = [zeros(3); eye(3)];
phi_k = [0; 0; dv ;
    [0; 0; 9.81]];
phi_k_apostroph = G*phi_k;
phi_k_apostroph = G*phi_k;

u1 =  -par(1) * sqrt(norm(sigma)) * sign(sigma);
%if abs(u) > par(6)
%    w =  - u;
%else
w = - par(2)*sign(sigma);
%end

== matlab function Controllers/SMC zero-order inner loops/CSMC/implicit euler ==
  data: x input double; u output double; sigma output double; tsim input double
function [u, sigma] = fcn(x, tsim)
coder.extrinsic('evalin');
coder.extrinsic('sandbox_extrinsic_zeroorder');
% G = zeros(1,2);
dt = 0;
a = zeros(1);
b = zeros(1);
% G = evalin('base', 'G');
a = evalin('base', 'a');
b = evalin('base', 'b');
dt = evalin('base', 'postracking.T');
G = [6 4];
%
% ueq = -(G*B)^-1*G*A*x;
%
sigma = G*x;

% Explicit:
udisc_expl = -sign(sigma);

% Implicit:
udisc_impl = 0;
if abs(sigma) <= dt
    udisc_impl =  - sigma/dt;
elseif sigma > dt
    udisc_impl = -1;
elseif sigma < -dt
    udisc_impl = 1;
end

u = 0;
u =  -1*udisc_expl;

if abs(sigma) <= 1e-1
 %   tic;
   %u = sandbox_extrinsic_zeroorder(x, G, dt, a, b);
%   toc
end

end

== matlab function Controllers/SMC zero-order inner loops/CSMC/MIMO STSMC/MATLAB Function ==
  data: u1 output double; dp input double; dv input double; da input double; w output double; sigma output double; u input double
function [u1, w, sigma ] = cstscm(dp, dv, da, u)
coder.extrinsic('cstscm_extrinsic');
coder.extrinsic('angle2dcm');
coder.extrinsic('evalin');

u1 = zeros(3,1);
w = zeros(3,1);
sigma = zeros(3,1);
N = zeros(3,1);

%[u1, w, sigma] = cstscm_extrinsic(dp, dv, da, u);

u1 = zeros(3,1);
w = zeros(3,1);
persistent lastsample;
if isempty(lastsample)
    lastsample.sigma = zeros(3,1);
    N = evalin('base', 'uavsim.svm.usat.n_c.upper')';
end

lp = [6 6 6];
lv = [4 4 4];
G = [diag(lp) diag(lv)];
sigma = G * [dp; dv];
lastsample.sigma = sigma;

% Compute controller in compliance with ACA article:
% Known disturbances:
B = [zeros(3); eye(3)];
phi_k = [dv;
    [0; 0; 9.81]];
phi_k_apostroph = G*phi_k;
upre = (1/9.81)*(G*B)^(-1)*phi_k_apostroph;

% Upper bounds on unknown disturbances:
Aw = [1 1 0.46 + 0.0083]';
%max load factors:
R_be = eye(3);
R_be = eye(3); %angle2dcm(0,0,0);
R_eb = R_be';
nc0 = R_be * [0 0 -1]';
U =  R_eb * 9.81 * (N - nc0);
apre_max = U;
phiu_max = Aw + apre_max;
phiuapostroph_max = G*B*phiu_max;
L = phiuapostroph_max;

% Run three SISO controllers:
for k=1:3
    alpha = 1.5*sqrt(L(k));
    beta = 1.1*L(k);
    u1(k) =   alpha * sqrt(norm(sigma(k))) * sign(sigma(k)) + upre(k);
    %if abs(u) > par(6)
    %    w =  - u;
    %else
    w(k) =  beta*sign(sigma(k));
    %end
end
end

== matlab function Controllers/SMC zero-order inner loops/DSMC/MIMO DSMC/MATLAB Function ==
  data: nc output double; dp input double; dv input double; da input double; sigma output double; ac input double; dbport output double; tsim input double
function [nc, sigma, dbport ] = dsmc(dp, dv, da, ac, tsim)
coder.extrinsic('dsmc_extrinsic');

nc = zeros(3,1);
sigma = zeros(3,1);
dbport = zeros(1,1);

[nc, sigma, dbport] = dsmc_extrinsic(dp, dv, da, ac, tsim);

end

== matlab function Load factor disturbances due to turbulence and wake/Wake disturbances/MATLAB Function ==
  data: nwake output double; dp input double
function nwake = nwakef(dp)
persistent b;
persistent m;
persistent c;
persistent CL_alpha;

coder.extrinsic('evalin');
coder.extrinsic('HSVM');
if isempty(b)
    b = evalin('base', 'uavsim.cularis.b');
    m = evalin('base', 'uavsim.cularis.mass');   
    c = evalin('base', 'uavsim.cularis.c');   
    CL_alpha = evalin('base', 'uavsim.cularis.CL_alpha');   
end

L = 9.81*m;
deltaL = 0;
deltaL = HSVM(dp, m, 15, 1.225, b, CL_alpha, c);

nwake = [0 0 deltaL/9.81]';
